simulink model "nid_cvst_pattern_matching"  (Simulink 7.8)
settings: Solver=FixedStepDiscrete  StartTime=0.0  StopTime=inf  RelTol=1e-3
undefined symbols (not defined in the file or in its folder): Rec, SDTV, strel
libraries: nid_lib x3, visiontextngfix x2, visionstatistics x1, visionconversions x1, simulink x1, visionmorphops x1, visionsinks x1
settings Model: Creator=nmaeda  LastModifiedBy=tchikama

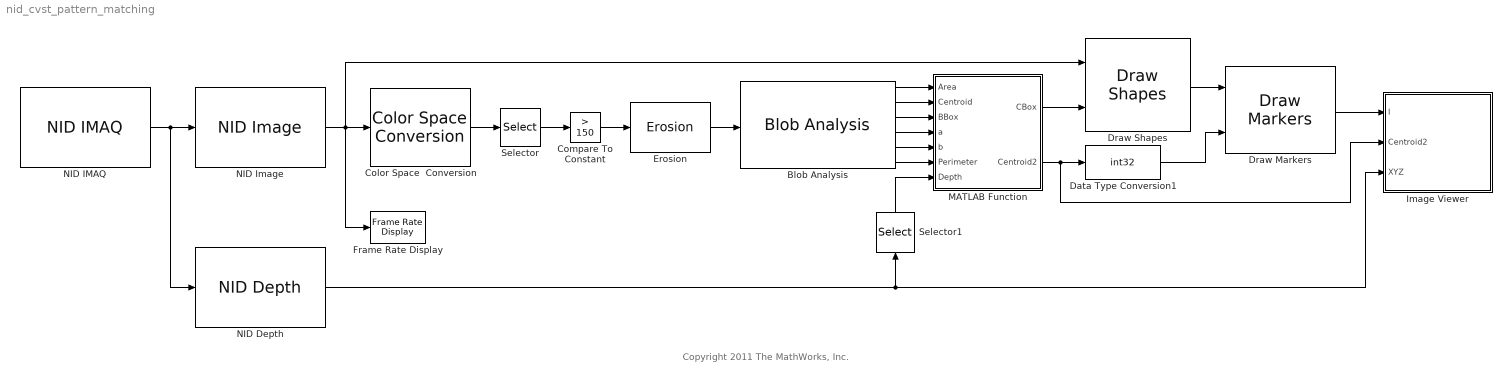
== system nid_cvst_pattern_matching ==
  note: Copyright 2011 The MathWorks, Inc.
  Blob Analysis : visionstatistics/Blob Analysis  Tag=vipblks_row_conv  area=on  centroid=on  bBox=on  majorAxis=on  minorAxis=on  angle=off  eccentricity=off  equivDiameterSq=off  extent=off  perimeter=on  maxBlobs=500  warnIfNumBlobsExceeded=on  isCount=off  useMinArea=off  minArea=0  useMaxArea=off  maxArea=intmax('uint32')  excludeBorderBlob=off  outDT=double  isOutVarDim=off  isFill=on  fillValues=-1  conn=8  isLabel=off  outputMode=Binary point scaling  outputWordLength=32  outputFracLength=16  firstCoeffMode=Binary point scaling  firstCoeffWordLength=16  firstCoeffFracLength=14  secondCoeffMode=Binary point scaling  secondCoeffWordLength=32  secondCoeffFracLength=16  accumMode=Binary point scaling  accumWordLength=32  accumFracLength=0  prodOutputMode=Binary point scaling  prodOutputWordLength=32  prodOutputFracLength=16  roundingMode=Floor  overflowMode=off
  Color Space  Conversion : visionconversions/Color Space  Conversion  conversion=Obsolete  conversionActive=R'G'B' to Y'CbCr  wp_str=D65  rec=Rec. 601 (SDTV)  sys=1125/60/2:1  imagePorts=One multidimensional signal
  Compare To Constant : simulink/Logic and Bit Operations/Compare To Constant  relop=>  const=150  OutDataTypeStr=boolean
  Data Type Conversion1 : DataTypeConversion  OutDataTypeStr=int32  RndMeth=Round
  Draw Markers : visiontextngfix/Draw Markers  shape=Star  size=3  fill=off  fillClrSource=Specify via dialog  display=User-specified value  intensity=155  color=[0 0 255]  opacity=0  viewport=Entire image  antialiasing=off  inType=Obsolete  imagePorts=One multidimensional signal  prodOutputMode=Binary point scaling  prodOutputWordLength=32  prodOutputFracLength=14  memoryMode=Specify word length  memoryWordLength=16  memoryFracLength=15  roundingMode=Floor  overflowMode=off
  Draw Shapes : visiontextngfix/Draw Shapes  shape=Rectangles  fill=off  fillClrSource=Specify via dialog  display=User-specified value  intensity=200  color=[0 0 255]  opacity=0.6  viewport=Entire image  antialiasing=off  inType=Obsolete  imagePorts=One multidimensional signal  prodOutputMode=Binary point scaling  prodOutputWordLength=32  prodOutputFracLength=14  memoryMode=Specify word length  memoryWordLength=16  memoryFracLength=15  roundingMode=Floor  overflowMode=off
  Erosion : visionmorphops/Erosion  nhoodsrc=Specify via dialog  strel=strel('square',4)
  Frame Rate Display : visionsinks/Frame Rate Display  UpdateRate=10
  Image Viewer : MATLAB Function  TreatAsAtomicUnit=on
  MATLAB Function : MATLAB Function  TreatAsAtomicUnit=on
  NID Depth : nid_lib/NID Depth  depthOutput=XYZ  conv_XYZ_RW=on  viewer=off
  NID IMAQ : nid_lib/NID IMAQ  imaq_depth=on  imaq_motion=off  imaq_image=on  view_point=on  imaq_skeleton=off  imaq_ir=off  mirror_image=off  res_fps=VGA (640x480): 30 FPS  imaq_sample_time=1/30
  NID Image : nid_lib/NID Image  imageOutput=RGB
  Selector : Selector  NumberOfDimensions=3  InputPortWidth=3  IndexOptions=Select all,Select all,Index vector (dialog)  Indices=[1 3],1,3  OutputSizes=1,1,1
  Selector1 : Selector  NumberOfDimensions=3  InputPortWidth=3  IndexOptions=Select all,Select all,Index vector (dialog)  Indices=[1 3],1,3  OutputSizes=1,1,1
  wires:
  Compare To Constant/1 -> Erosion/1
  NID IMAQ/1 -> NID Image/1, NID Depth/1
  MATLAB Function/1(CBox) -> Draw Shapes/2
  NID Image/1 -> Draw Shapes/1, Color Space  Conversion/1, Frame Rate Display/1
  Erosion/1 -> Blob Analysis/1
  Blob Analysis/1 -> MATLAB Function/1(Area)
  Blob Analysis/2 -> MATLAB Function/2(Centroid)
  Blob Analysis/3 -> MATLAB Function/3(BBox)
  Blob Analysis/4 -> MATLAB Function/4(a)
  Blob Analysis/5 -> MATLAB Function/5(b)
  Blob Analysis/6 -> MATLAB Function/6(Perimeter)
  NID Depth/1 -> Image Viewer/3(XYZ), Selector1/1
  Color Space  Conversion/1 -> Selector/1
  Selector/1 -> Compare To Constant/1
  MATLAB Function/2(Centroid2) -> Data Type Conversion1/1, Image Viewer/2(Centroid2)
  Draw Shapes/1 -> Draw Markers/1
  Data Type Conversion1/1 -> Draw Markers/2
  Draw Markers/1 -> Image Viewer/1(I)
  Selector1/1 -> MATLAB Function/7(Depth)

== matlab function Image Viewer ==
  data: I input double; Centroid2 input double; XYZ input double
function fcn(I, Centroid2, XYZ)
%#codegen

coder.extrinsic('image');
coder.extrinsic('axis');
coder.extrinsic('text');
coder.extrinsic('hold');
coder.extrinsic('num2str');
coder.extrinsic('drawnow');

m = size(Centroid2,1);
image(I);
axis off;
for n = 1:m
    if Centroid2(n,1)~=-1;
        X = round(Centroid2(n,1));
        Y = round(Centroid2(n,2));
        hold('on');
        text(X,Y,['  ','X:',num2str(XYZ(Y,X,1),3),' Y:',num2str(XYZ(Y,X,2),3),' Z:',num2str(XYZ(Y,X,3),3)]);
        hold('off');
    end
end
drawnow;

== matlab function MATLAB Function ==
  data: Area input double; Centroid input double; BBox input double; a input double; CBox output double; Centroid2 output double; b input double; Perimeter input double; Depth input double
function [CBox,Centroid2] = fcn(Area, Centroid, BBox, a, b, Perimeter, Depth)
%#codegen

m = length(a);
Ptemp = zeros(m,1);
Rate = zeros(m,1);
CBox = BBox;
a=0.5.*a;
b=0.5.*b;
Th = 150;

for n = 1:m
    Ptemp(n) = pi.*sqrt(2.*(a(n).^2+b(n).^2)-(a(n)-b(n)).^2./2.2);
    Rate(n) = Ptemp(n)./Perimeter(n);
    if Ptemp(n)./Perimeter(n)>1.1 || Ptemp(n)./Perimeter(n)<0.9
        CBox(n,:)=-1;
    end
    if Area(n)<Th
        CBox(n,:)=-1;
    end
    
    X = round(Centroid(n,1));
    Y = round(Centroid(n,2));
    if X>0 || Y > 0
        if Depth(Y,X)==0 || Depth(Y,X)>2
            CBox(n,:)=-1;
        end
    end    
end

Centroid2 = Centroid;
for n = 1:m
    if CBox(n,1)==-1
        Centroid2(n,:)=-1;   
    end
end
